simulink library "idlib"  (Simulink 5.1)
libraries: simulink_extras x2, simulink x1
settings Model: LastModifiedBy=LaoYU  ProdHWDeviceType=Microprocessor

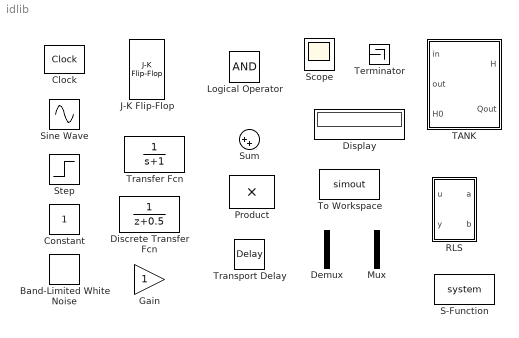
== system idlib ==
  Band-Limited White Noise : simulink/Sources/Band-Limited White Noise  Cov=[0.1]  Ts=0.1  seed=[23341]
  Clock : simulink_extras/Flip Flops/Clock  MaskParam1=2
  Constant : Constant
  Demux : Demux  Outputs=2
  Discrete Transfer Fcn : DiscreteTransferFcn
  Display : Display
  Gain : Gain  SaturateOnIntegerOverflow=on
  J-K Flip-Flop : simulink_extras/Flip Flops/J-K Flip-Flop  initial_condition=0
  Logical Operator : Logic  AllPortsSameDT=off
  Mux : Mux  Inputs=2
  Product : Product  SaturateOnIntegerOverflow=on
  RLS : Subsystem  mask(递推最小二乘法辨识模块){nn=2, lmd=1, Ts=1}
      mask prompts: nn "模型阶次"; lmd "遗忘因子(0.9～1)"; Ts "采样周期"
      mask help: 　　采用带有遗忘因子的递推最小二乘法估计模型参数。 　　模型的阶次：差分方程模型的阶次； 　　遗忘因子：用于辨识时变系统模型，定常系统取1； 　　采样周期：模型的采样周期。
      mask Help: RLS
      mask Display: disp('RLS')
  S-Function : S-Function
  Scope : Scope
  Sine Wave : Sin  SampleTime=0
  Step : Step  SampleTime=0
  Sum : Sum  Inputs=|++  SaturateOnIntegerOverflow=on
  TANK : Subsystem  mask(水罐液位流量模块){A=50, Kin=2, Kout=30, Ts=-1}
      mask prompts: A "水罐截面积A"; Kin "进水管道流量系数Kin"; Kout "出水管道流量系数Kout"; Ts "计算步长"
      mask help:
      | Adh/dt=Kin*u1-Kout*u2*Sqrt(h-u3)
      |     y1=h
      |     y2=Qout
      mask Help: 使用该模块可以构造多个水罐串联或并联的系统，模型为机理非线性模型。
      mask Display:
      | plot([0,0,10,10,0],[0,10,10,0,0],[0,10],[7,7],[2,8],[6,6],[4,6],[5,5]);
      | port_label('output', 1, 'H ');
      | port_label('output', 2, 'Qo ');
      | port_label('input', 1, ' U1');
      | port_label('input', 2, ' U2');
      | port_label('input', 3, ' Ho');
  Terminator : Terminator
  To Workspace : ToWorkspace  VariableName=simout  SampleTime=-1  SaveFormat=Structure
  Transfer Fcn : TransferFcn  Denominator=[1 1]
  Transport Delay : TransportDelay

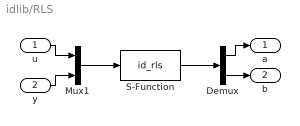
== system idlib/RLS ==
  u : Inport
  y : Inport  Port=2
  Demux : Demux  Outputs=[nn nn]
  Mux1 : Mux  Inputs=2
  S-Function : S-Function  FunctionName=id_rls  Parameters=nn,lmd,Ts
  a : Outport
  b : Outport  Port=2
  wires:
  Mux1/1 -> S-Function/1
  S-Function/1 -> Demux/1
  Demux/1 -> a/1
  u/1 -> Mux1/1
  Demux/2 -> b/1
  y/1 -> Mux1/2

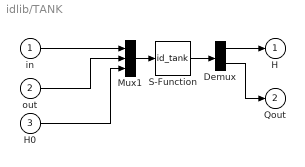
== system idlib/TANK ==
  in : Inport
  out : Inport  Port=2
  H0 : Inport  Port=3
  Demux : Demux  Outputs=2
  Mux1 : Mux  Inputs=3
  S-Function : S-Function  FunctionName=id_tank  Parameters=A, Kin,Kout,Ts
  H : Outport
  Qout : Outport  Port=2
  wires:
  H0/1 -> Mux1/3
  Demux/2 -> Qout/1
  Demux/1 -> H/1
  S-Function/1 -> Demux/1
  in/1 -> Mux1/1
  out/1 -> Mux1/2
  Mux1/1 -> S-Function/1
